simulink model "test_lookup_table"  (R2025b)
settings: Solver=FixedStepAuto  StartTime=0.0  StopTime=25  FixedStep=10e-5  RelTol=1e-3
values from neighbouring files (symbols this model uses):
  repos_actionneur = deplacement_statique(idx_force_reduit)    [lookup_table_statespace.m]
libraries: cstblocks x1
settings Model: Creator=FV  LastModifiedBy=FV

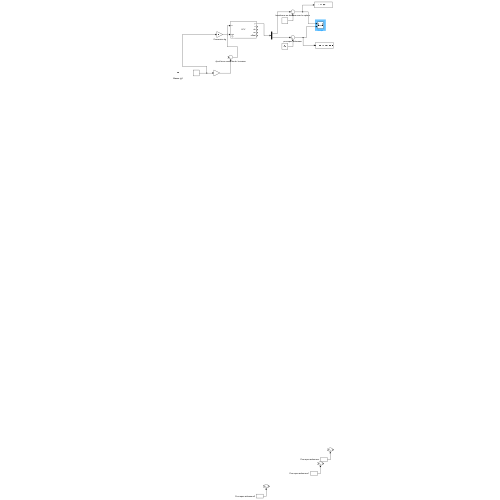
[thumbnail: Simulink's stored preview of the top-level diagram]
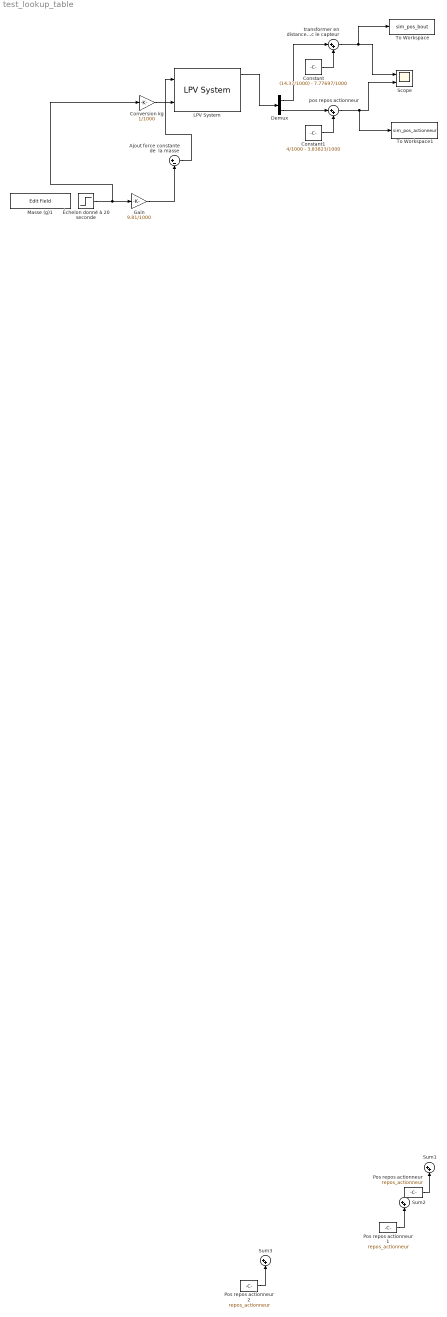
== system test_lookup_table ==
  Ajout force constante de  la masse : Sum  Inputs=|+-
  Constant : Constant  Value=(14.37/1000) - 7.77697/1000
  Constant1 : Constant  Value=4/1000 - 3.83823/1000
  Conversion kg : Gain  Gain=1/1000
  Demux : Demux  Outputs=2
  Gain : Gain  Gain=9.81/1000
  LPV System : cstblocks/Linear Parameter Varying/LPV System  sys=sys_array  InitialConditionSource=internal  InitialCondition=0  opSpecOption=Specify offsets as double arrays  uOffset=0  yOffset=0  xOffset=0  opEquilOption=on  dxOffset=0  AFixed=false  BFixed=false  CFixed=false  DFixed=false  uDelayFixed=false  yDelayFixed=false  iDelayFixed=false  sysFixedOption=First model in state-space array  sysFixed=[]  IMethod=Linear  EMethod=Clip  IndexSearch=Binary search  IndexBegin=on  OutputX=on  OutputXdot=on  OutputLTI=on  OutputOP=on  DataType=double  InitBufferSize=1024  FixedBuffer=off  SimMode=Interpreted execution  Offset=struct
  Masse (g)1 : EditField  LabelPosition=Hide  ShowInitialText=on  Alignment=Center
  Pos repos actionneur : Constant  Value=repos_actionneur
  Pos repos actionneur1 : Constant  Value=repos_actionneur
  Pos repos actionneur2 : Constant  Value=repos_actionneur
  Scope : Scope  NumInputPorts=2
      settings: ActiveDisplayYMinimum=-0.0029844003484171167  ActiveDisplayYMaximum=0.0076608004479152081
  Sum1 : Sum  Inputs=|++
  Sum2 : Sum  Inputs=|++
  Sum3 : Sum  Inputs=|++
  To Workspace : ToWorkspace  VariableName=sim_pos_bout  SampleTime=-1
  To Workspace1 : ToWorkspace  VariableName=sim_pos_actionneur  SampleTime=-1
  pos repos actionneur : Sum  Inputs=|++
  transformer en distance avec le capteur : Sum  Inputs=|++
  Échelon donné à 20 seconde : Step  Time=20  After=50  SampleTime=0
  wires:
  Échelon donné à 20 seconde/1 -> Gain/1, Conversion kg/1
  Gain/1 -> Ajout force constante de  la masse/2
  Conversion kg/1 -> LPV System/2
  Ajout force constante de  la masse/1 -> LPV System/1
  LPV System/1 -> Demux/1
  Pos repos actionneur/1 -> Sum1/2
  Pos repos actionneur1/1 -> Sum2/2
  Pos repos actionneur2/1 -> Sum3/2
  transformer en distance avec le capteur/1 -> To Workspace/1, Scope/1
  Demux/1 -> transformer en distance avec le capteur/1
  Demux/2 -> pos repos actionneur/1
  pos repos actionneur/1 -> To Workspace1/1, Scope/2
  Constant1/1 -> pos repos actionneur/2
  Constant/1 -> transformer en distance avec le capteur/2
